simulink model "Prueba_boggieDynamics"  (R2022b)
settings: Solver=VariableStepAuto  StartTime=0.0  StopTime=5  RelTol=1e-3
InitFcn:
  | m = 200;
  | g = 9.81;
  | Ixx = 12.489414;
  | Iyy = 52.598747;
  | Izz = 53.106596;
  | 
  | x_lev12 = 1;
  | x_lev34 = 1;
  | x_lim = 0.1;
  | 
  | y_lev13 = 1;
  | y_lev24 = 1;
  | y_lim = 0.1;
  | y_brk = 0.1;
  | 
  | z_lev = 1;
  | z_lim = 0.1;
  | z_brk = 0.1;
  | 
  | cg_nom = 0.3;
  | 
  | I = [2 1 1;1 2 1 ;1 1 2 ]
  | %I2 = [-0.0117539 0.116439 12.4897 ; -0.0021666 52.5984 0.116439;  53.10658 -0.00216668 -0.0117539]
libraries: shared6dof x1
settings Model: Creator=USUARIO  LastModifiedBy=USUARIO

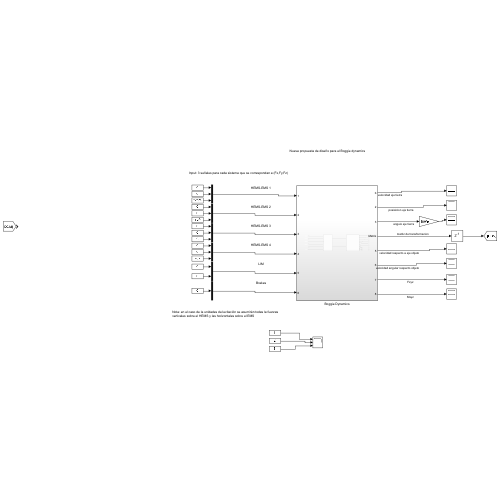
[thumbnail: Simulink's stored preview of the top-level diagram]
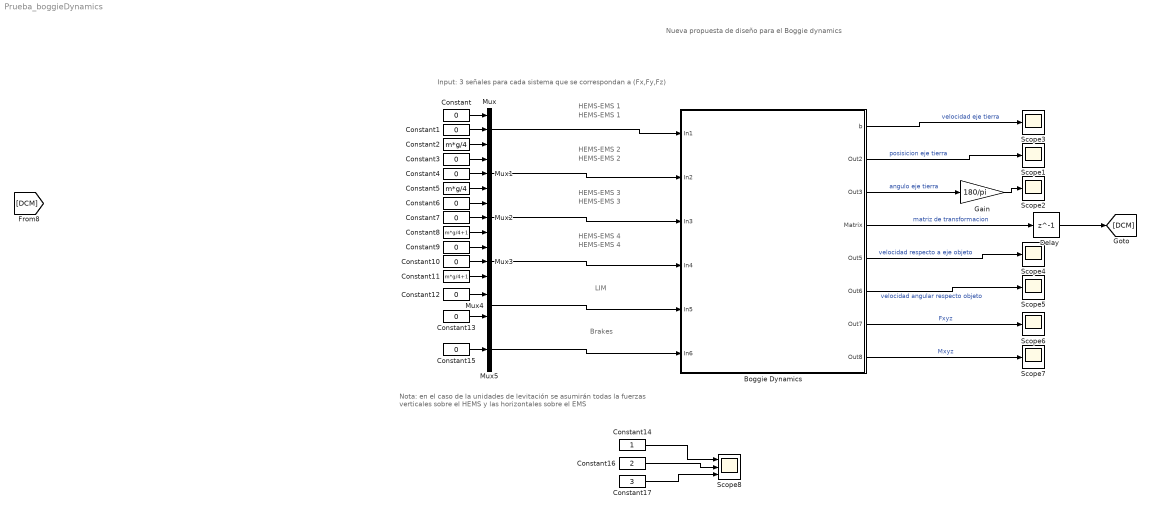
== system Prueba_boggieDynamics ==
  note: Input: 3 señales para cada sistema que se correspondan a (Fx,Fy,Fz)
  note: Nueva propuesta de diseño para el Boggie dynamics
  note: HEMS-EMS 3
  note: Brakes
  note: HEMS-EMS 1
  note: LIM
  note: HEMS-EMS 4
  note: HEMS-EMS 2
  note: Nota: en el caso de la unidades de levitación se asumirán todas la fuerzas
      | verticales sobre el HEMS y las horizontales sobre el EMS
  note: HEMS-EMS 1
  note: HEMS-EMS 2
  note: HEMS-EMS 4
  note: HEMS-EMS 3
  Boggie Dynamics : Subsystem
  Constant{,1,3..4,6..7,9..10,12..13,15} (11 alike) : Constant  Value=0
  Constant11 : Constant  Value=m*g/4+1
  Constant14 : Constant
  Constant16 : Constant  Value=2
  Constant17 : Constant  Value=3
  Constant2 : Constant  Value=m*g/4
  Constant5 : Constant  Value=m*g/4
  Constant8 : Constant  Value=m*g/4+1
  Delay : Delay  DelayLength=1
  Gain : Gain  Gain=180/pi
  Mux{,1..3} (4 alike) : Mux  Inputs=3
  Mux4 : Mux  Inputs=2
  Mux5 : Mux  Inputs=1
  Scope{1..7} (7 alike) : Scope
  Scope8 : Scope  NumInputPorts=3
  wires:
  Boggie Dynamics/2(Out2) -> Scope1/1  "posisicion eje tierra"
  Boggie Dynamics/3(Out3) -> Gain/1  "angulo eje tierra"
  Boggie Dynamics/1(b) -> Scope3/1  "velocidad eje tierra"
  Constant1/1 -> Mux/2
  Constant/1 -> Mux/1
  Constant3/1 -> Mux1/1
  Constant4/1 -> Mux1/2
  Constant6/1 -> Mux2/1
  Constant8/1 -> Mux2/3
  Constant7/1 -> Mux2/2
  Constant9/1 -> Mux3/1
  Constant11/1 -> Mux3/3
  Constant10/1 -> Mux3/2
  Constant12/1 -> Mux4/1
  Constant13/1 -> Mux4/2
  Constant15/1 -> Mux5/1
  Boggie Dynamics/6(Out6) -> Scope5/1  "velocidad angular respecto objeto"
  Boggie Dynamics/4(Matrix) -> Delay/1  "matriz de transformacion"
  Boggie Dynamics/5(Out5) -> Scope4/1  "velocidad respecto a eje objeto"
  Boggie Dynamics/8(Out8) -> Scope7/1  "Mxyz"
  Boggie Dynamics/7(Out7) -> Scope6/1  "Fxyz"
  Constant14/1 -> Scope8/1
  Constant16/1 -> Scope8/2
  Constant17/1 -> Scope8/3
  Gain/1 -> Scope2/1
  Constant2/1 -> Mux/3
  Constant5/1 -> Mux1/3
  Mux2/1 -> Boggie Dynamics/3(In3)
  Mux3/1 -> Boggie Dynamics/4(In4)
  Mux/1 -> Boggie Dynamics/1(In1)
  Mux1/1 -> Boggie Dynamics/2(In2)
  Mux4/1 -> Boggie Dynamics/5(In5)
  Mux5/1 -> Boggie Dynamics/6(In6)
  Delay/1 -> [DCM]

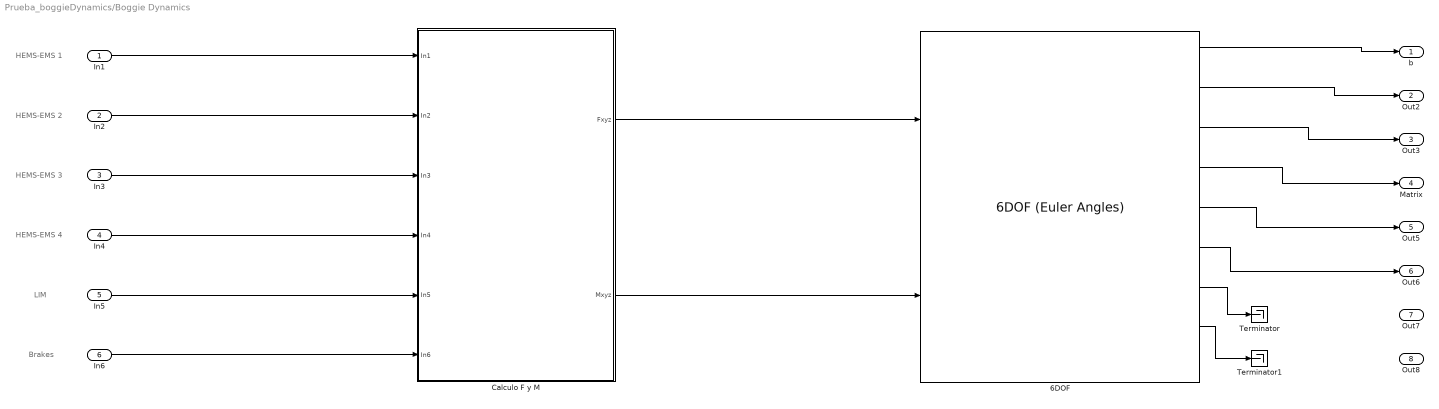
== system Prueba_boggieDynamics/Boggie Dynamics ==
  note: LIM
  note: HEMS-EMS 1
  note: HEMS-EMS 2
  note: HEMS-EMS 3
  note: HEMS-EMS 4
  note: Brakes
  In1 : Inport
  In2 : Inport  Port=2
  In3 : Inport  Port=3
  In4 : Inport  Port=4
  In5 : Inport  Port=5
  In6 : Inport  Port=6
  "6DOF " : shared6dof/6DOF (Euler Angles)  units=Metric (MKS)  mtype=Fixed  rep=Euler Angles  xme_0=[0 0 cg_nom]  Vm_0=[0 0 0]  eul_0=[0 0.5 0]  pm_0=[0 0 0]  mass_0=m  mass_e=0.5  mass_f=2.0  inertia=I  inertia_e=eye(3)  inertia_f=2*eye(3)  k_quat=1.0  vre_flag=on  abi_flag=on  aMode=0  xme_statename=''  Vm_statename=''  eul_statename=''  quat_statename=''  pm_statename=''  mass_statename=''
  Calculo F y M : Subsystem
  Terminator : Terminator
  Terminator1 : Terminator
  b : Outport
  Out2 : Outport  Port=2
  Out3 : Outport  Port=3
  Matrix : Outport  Port=4
  Out5 : Outport  Port=5
  Out6 : Outport  Port=6
  Out7 : Outport  Port=7
  Out8 : Outport  Port=8
  wires:
  "6DOF "/1 -> b/1
  "6DOF "/2 -> Out2/1
  "6DOF "/3 -> Out3/1
  In1/1 -> Calculo F y M/1(In1)
  In2/1 -> Calculo F y M/2(In2)
  In3/1 -> Calculo F y M/3(In3)
  In4/1 -> Calculo F y M/4(In4)
  In5/1 -> Calculo F y M/5(In5)
  In6/1 -> Calculo F y M/6(In6)
  Calculo F y M/1(Fxyz) -> "6DOF "/1
  "6DOF "/5 -> Out5/1
  "6DOF "/6 -> Out6/1
  "6DOF "/8 -> Terminator1/1
  "6DOF "/7 -> Terminator/1
  Calculo F y M/2(Mxyz) -> "6DOF "/2
  "6DOF "/4 -> Matrix/1

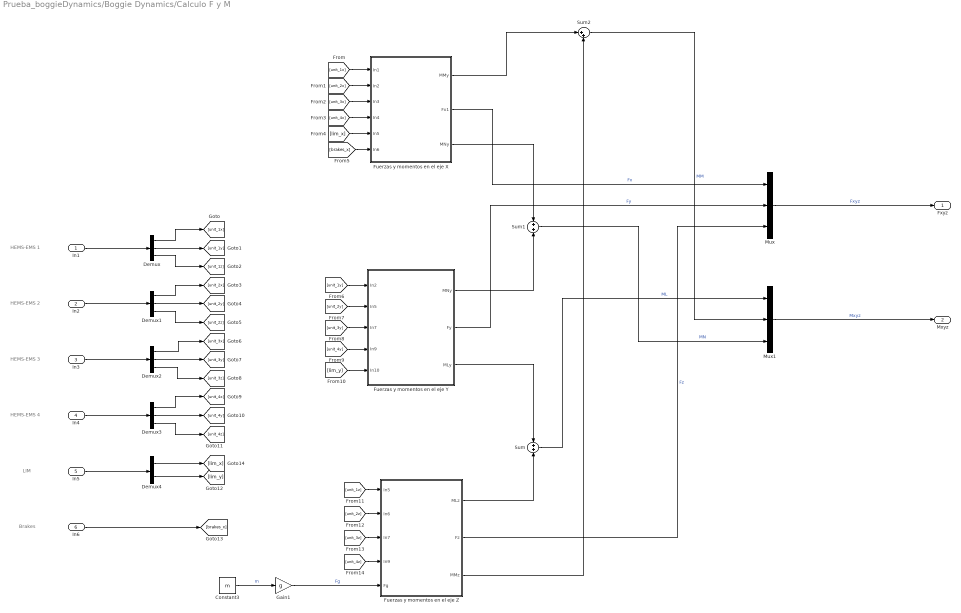
== system Prueba_boggieDynamics/Boggie Dynamics/Calculo F y M ==
  note: HEMS-EMS 3
  note: Brakes
  note: HEMS-EMS 1
  note: LIM
  note: HEMS-EMS 4
  note: HEMS-EMS 2
  In1 : Inport
  In2 : Inport  Port=2
  In3 : Inport  Port=3
  In4 : Inport  Port=4
  In5 : Inport  Port=5
  In6 : Inport  Port=6
  Constant3 : Constant  Value=m
  Demux{,1..3} (4 alike) : Demux  Outputs=3
  Demux4 : Demux  Outputs=2
  Fuerzas y momentos en el eje X : Subsystem
  Fuerzas y momentos en el eje Y : Subsystem
  Fuerzas y momentos en el eje Z : Subsystem
  Gain1 : Gain  Gain=g
  Mux : Mux  Inputs=3
  Mux1 : Mux  Inputs=3
  Sum : Sum
  Sum1 : Sum
  Sum2 : Sum  Inputs=|++
  Fxyz : Outport
  Mxyz : Outport  Port=2
  wires:
  In3/1 -> Demux2/1
  Constant3/1 -> Gain1/1  "m"
  Sum2/1 -> Mux1/2  "MM"
  Mux/1 -> Fxyz/1  "Fxyz"
  In4/1 -> Demux3/1
  Mux1/1 -> Mxyz/1  "Mxyz"
  Sum1/1 -> Mux1/3  "MN"
  Sum/1 -> Mux1/1  "ML"
  In2/1 -> Demux1/1
  In5/1 -> Demux4/1
  In6/1 -> [brakes_x]
  In1/1 -> Demux/1
  Fuerzas y momentos en el eje X/1(MMy) -> Sum2/1
  Fuerzas y momentos en el eje X/2(Fx1) -> Mux/1  "Fx"
  Fuerzas y momentos en el eje X/3(MNy) -> Sum1/1
  Fuerzas y momentos en el eje Y/2(Fy) -> Mux/2  "Fy"
  Fuerzas y momentos en el eje Y/1(MNy) -> Sum1/2
  Fuerzas y momentos en el eje Y/3(MLy) -> Sum/1
  Gain1/1 -> Fuerzas y momentos en el eje Z/5(Fg)  "Fg"
  Fuerzas y momentos en el eje Z/2(Fz) -> Mux/3  "Fz"
  Fuerzas y momentos en el eje Z/1(MLz) -> Sum/2
  Demux4/2 -> [lim_y]
  Demux4/1 -> [lim_x]
  Demux3/1 -> [unit_4x]
  Demux3/2 -> [unit_4y]
  Demux3/3 -> [unit_4z]
  Demux2/1 -> [unit_3x]
  Demux2/2 -> [unit_3y]
  Demux2/3 -> [unit_3z]
  Demux1/1 -> [unit_2x]
  Demux1/2 -> [unit_2y]
  Demux1/3 -> [unit_2z]
  Demux/1 -> [unit_1x]
  Demux/2 -> [unit_1y]
  Demux/3 -> [unit_1z]
  [unit_1x] -> Fuerzas y momentos en el eje X/1(In1)
  [unit_2x] -> Fuerzas y momentos en el eje X/2(In2)
  [unit_3x] -> Fuerzas y momentos en el eje X/3(In3)
  [unit_4x] -> Fuerzas y momentos en el eje X/4(In4)
  [lim_x] -> Fuerzas y momentos en el eje X/5(In5)
  [brakes_x] -> Fuerzas y momentos en el eje X/6(In6)
  [unit_4y] -> Fuerzas y momentos en el eje Y/4(In9)
  [unit_1y] -> Fuerzas y momentos en el eje Y/1(In2)
  [lim_y] -> Fuerzas y momentos en el eje Y/5(In10)
  [unit_2y] -> Fuerzas y momentos en el eje Y/2(In5)
  [unit_3y] -> Fuerzas y momentos en el eje Y/3(In7)
  [unit_1z] -> Fuerzas y momentos en el eje Z/1(In5)
  [unit_3z] -> Fuerzas y momentos en el eje Z/3(In7)
  [unit_2z] -> Fuerzas y momentos en el eje Z/2(In6)
  [unit_4z] -> Fuerzas y momentos en el eje Z/4(In9)
  Fuerzas y momentos en el eje Z/3(MMz) -> Sum2/2

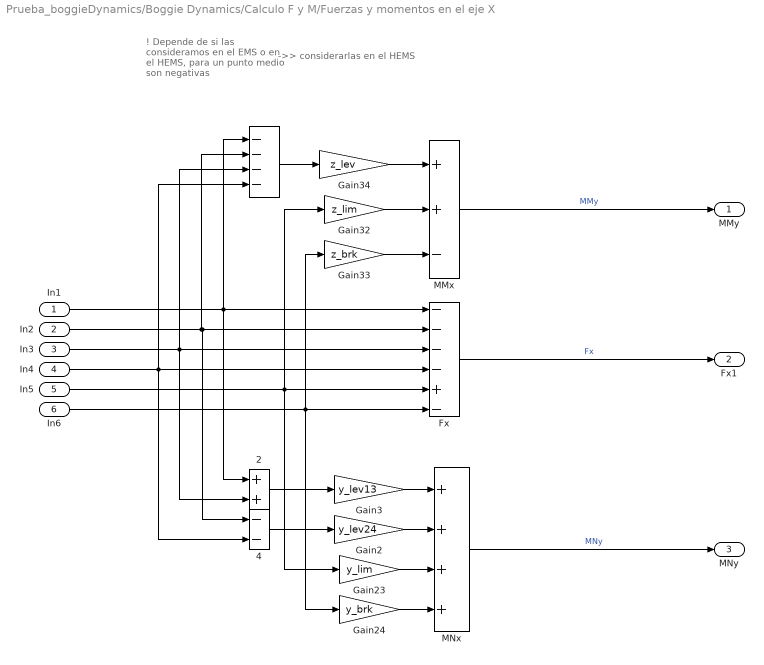
== system Prueba_boggieDynamics/Boggie Dynamics/Calculo F y M/Fuerzas y momentos en el eje X ==
  note: ! Depende de si las consideramos en el EMS o en el HEMS,
      | para un punto medio son negativas
  note: ->> considerarlas en el HEMS
  In1 : Inport
  In2 : Inport  Port=2
  In3 : Inport  Port=3
  In4 : Inport  Port=4
  In5 : Inport  Port=5
  In6 : Inport  Port=6
  " " : Sum  Inputs=----
  " 2" : Sum
  " 4" : Sum  Inputs=--
  Fx : Sum  Inputs=----+-
  Gain2 : Gain  Gain=y_lev24
  Gain23 : Gain  Gain=y_lim
  Gain24 : Gain  Gain=y_brk
  Gain3 : Gain  Gain=y_lev13
  Gain32 : Gain  Gain=z_lim
  Gain33 : Gain  Gain=z_brk
  Gain34 : Gain  Gain=z_lev
  MMx : Sum  Inputs=++-
  MNx : Sum  Inputs=++++
  MMy : Outport
  Fx1 : Outport  Port=2
  MNy : Outport  Port=3
  wires:
  In1/1 -> " 2"/1, " "/1, Fx/1
  In2/1 -> " "/2, " 4"/1, Fx/2
  Fx/1 -> Fx1/1  "Fx"
  MMx/1 -> MMy/1  "MMy"
  In4/1 -> " 4"/2, " "/4, Fx/4
  In6/1 -> Gain24/1, Fx/6, Gain33/1
  In5/1 -> Fx/5, Gain23/1, Gain32/1
  In3/1 -> " "/3, " 2"/2, Fx/3
  Gain32/1 -> MMx/2
  Gain34/1 -> MMx/1
  Gain33/1 -> MMx/3
  MNx/1 -> MNy/1  "MNy"
  " "/1 -> Gain34/1
  Gain24/1 -> MNx/4
  Gain23/1 -> MNx/3
  " 4"/1 -> Gain2/1
  " 2"/1 -> Gain3/1
  Gain3/1 -> MNx/1
  Gain2/1 -> MNx/2

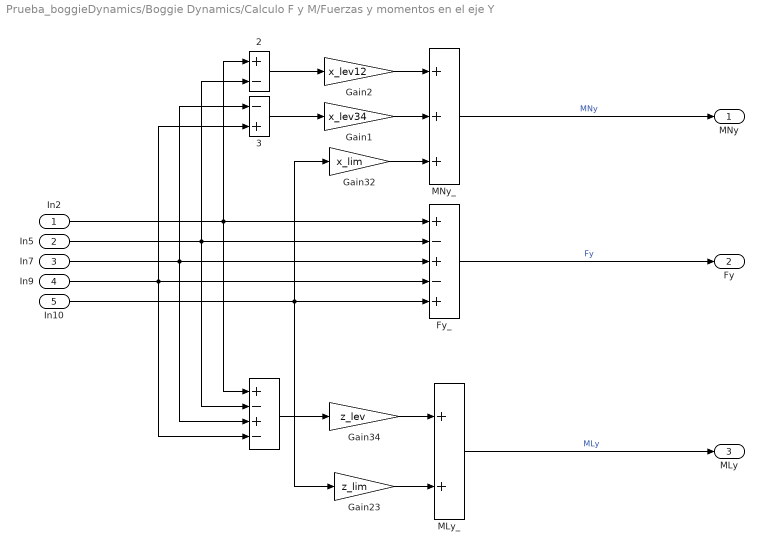
== system Prueba_boggieDynamics/Boggie Dynamics/Calculo F y M/Fuerzas y momentos en el eje Y ==
  In2 : Inport
  In5 : Inport  Port=2
  In7 : Inport  Port=3
  In9 : Inport  Port=4
  In10 : Inport  Port=5
  " " : Sum  Inputs=+-+-
  " 2" : Sum  Inputs=+-
  " 3" : Sum  Inputs=-+
  Fy_ : Sum  Inputs=+-+-+
  Gain1 : Gain  Gain=x_lev34
  Gain2 : Gain  Gain=x_lev12
  Gain23 : Gain  Gain=z_lim
  Gain32 : Gain  Gain=x_lim
  Gain34 : Gain  Gain=z_lev
  MLy_ : Sum
  MNy_ : Sum  Inputs=+++
  MNy : Outport
  Fy : Outport  Port=2
  MLy : Outport  Port=3
  wires:
  Fy_/1 -> Fy/1  "Fy"
  MLy_/1 -> MLy/1  "MLy"
  Gain32/1 -> MNy_/3
  In7/1 -> Fy_/3, " "/3, " 3"/1
  In9/1 -> " "/4, " 3"/2, Fy_/4
  In2/1 -> " "/1, " 2"/1, Fy_/1
  In5/1 -> " "/2, Fy_/2, " 2"/2
  MNy_/1 -> MNy/1  "MNy"
  In10/1 -> Gain32/1, Gain23/1, Fy_/5
  Gain23/1 -> MLy_/2
  " 3"/1 -> Gain1/1
  " 2"/1 -> Gain2/1
  Gain1/1 -> MNy_/2
  Gain2/1 -> MNy_/1
  " "/1 -> Gain34/1
  Gain34/1 -> MLy_/1

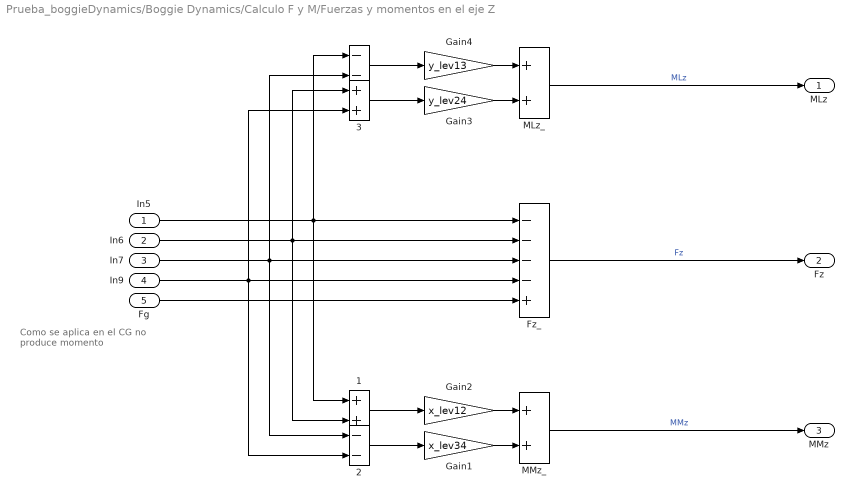
== system Prueba_boggieDynamics/Boggie Dynamics/Calculo F y M/Fuerzas y momentos en el eje Z ==
  note: Como se aplica en el CG
      |  no produce momento
  In5 : Inport
  In6 : Inport  Port=2
  In7 : Inport  Port=3
  In9 : Inport  Port=4
  Fg : Inport  Port=5
  " " : Sum  Inputs=--
  " 1" : Sum
  " 2" : Sum  Inputs=--
  " 3" : Sum
  " MLz_" : Sum
  " MMz_" : Sum
  Fz_ : Sum  Inputs=----+
  Gain1 : Gain  Gain=x_lev34
  Gain2 : Gain  Gain=x_lev12
  Gain3 : Gain  Gain=y_lev24
  Gain4 : Gain  Gain=y_lev13
  MLz : Outport
  Fz : Outport  Port=2
  MMz : Outport  Port=3
  wires:
  In6/1 -> " 1"/2, Fz_/2, " 3"/1
  " MLz_"/1 -> MLz/1  "MLz"
  Fg/1 -> Fz_/5
  In9/1 -> Fz_/4, " 2"/2, " 3"/2
  In5/1 -> " 1"/1, " "/1, Fz_/1
  In7/1 -> " 2"/1, Fz_/3, " "/2
  Fz_/1 -> Fz/1  "Fz"
  " MMz_"/1 -> MMz/1  "MMz"
  " 3"/1 -> Gain3/1
  " "/1 -> Gain4/1
  Gain4/1 -> " MLz_"/1
  Gain3/1 -> " MLz_"/2
  Gain2/1 -> " MMz_"/1
  " 2"/1 -> Gain1/1
  Gain1/1 -> " MMz_"/2
  " 1"/1 -> Gain2/1
